simulink model "sudoku"  (R2012b)
settings: Solver=ode45  StartTime=0.0  StopTime=10.0  RelTol=1e-3
libraries: sldvlib x83
(part 2 of 4)

== system sudoku/bounds2 ==
  In1 : Inport
  Assumption : sldvlib/Objectives and Constraints/Assumption  enabled=on  customAVTBlockType=Assumption  intervals=true  initial=off  dispValues=on  outEnabled=on
      settings: AttributesFormatString=%<intervals>
  Logical Operator : Logic  AllPortsSameDT=off  OutDataTypeStr=boolean
  geq : RelationalOperator  Operator=<=  OutDataTypeStr=boolean
  lb : Constant  OutDataTypeStr=int8
  leq : RelationalOperator  Operator=<=  OutDataTypeStr=boolean
  ub : Constant  Value=9  OutDataTypeStr=int8
  wires:
  In1/1 -> geq/1, leq/2
  geq/1 -> Logical Operator/2
  ub/1 -> geq/2
  leq/1 -> Logical Operator/1
  Logical Operator/1 -> Assumption/1
  lb/1 -> leq/1

== system sudoku/bounds20 ==
  In1 : Inport
  Assumption : sldvlib/Objectives and Constraints/Assumption  enabled=on  customAVTBlockType=Assumption  intervals=true  initial=off  dispValues=on  outEnabled=on
      settings: AttributesFormatString=%<intervals>
  Logical Operator : Logic  AllPortsSameDT=off  OutDataTypeStr=boolean
  geq : RelationalOperator  Operator=<=  OutDataTypeStr=boolean
  lb : Constant  OutDataTypeStr=int8
  leq : RelationalOperator  Operator=<=  OutDataTypeStr=boolean
  ub : Constant  Value=9  OutDataTypeStr=int8
  wires:
  In1/1 -> geq/1, leq/2
  geq/1 -> Logical Operator/2
  ub/1 -> geq/2
  leq/1 -> Logical Operator/1
  Logical Operator/1 -> Assumption/1
  lb/1 -> leq/1

== system sudoku/bounds21 ==
  In1 : Inport
  Assumption : sldvlib/Objectives and Constraints/Assumption  enabled=on  customAVTBlockType=Assumption  intervals=true  initial=off  dispValues=on  outEnabled=on
      settings: AttributesFormatString=%<intervals>
  Logical Operator : Logic  AllPortsSameDT=off  OutDataTypeStr=boolean
  geq : RelationalOperator  Operator=<=  OutDataTypeStr=boolean
  lb : Constant  OutDataTypeStr=int8
  leq : RelationalOperator  Operator=<=  OutDataTypeStr=boolean
  ub : Constant  Value=9  OutDataTypeStr=int8
  wires:
  In1/1 -> geq/1, leq/2
  geq/1 -> Logical Operator/2
  ub/1 -> geq/2
  leq/1 -> Logical Operator/1
  Logical Operator/1 -> Assumption/1
  lb/1 -> leq/1

== system sudoku/bounds22 ==
  In1 : Inport
  Assumption : sldvlib/Objectives and Constraints/Assumption  enabled=on  customAVTBlockType=Assumption  intervals=true  initial=off  dispValues=on  outEnabled=on
      settings: AttributesFormatString=%<intervals>
  Logical Operator : Logic  AllPortsSameDT=off  OutDataTypeStr=boolean
  geq : RelationalOperator  Operator=<=  OutDataTypeStr=boolean
  lb : Constant  OutDataTypeStr=int8
  leq : RelationalOperator  Operator=<=  OutDataTypeStr=boolean
  ub : Constant  Value=9  OutDataTypeStr=int8
  wires:
  In1/1 -> geq/1, leq/2
  geq/1 -> Logical Operator/2
  ub/1 -> geq/2
  leq/1 -> Logical Operator/1
  Logical Operator/1 -> Assumption/1
  lb/1 -> leq/1

== system sudoku/bounds23 ==
  In1 : Inport
  Assumption : sldvlib/Objectives and Constraints/Assumption  enabled=on  customAVTBlockType=Assumption  intervals=true  initial=off  dispValues=on  outEnabled=on
      settings: AttributesFormatString=%<intervals>
  Logical Operator : Logic  AllPortsSameDT=off  OutDataTypeStr=boolean
  geq : RelationalOperator  Operator=<=  OutDataTypeStr=boolean
  lb : Constant  OutDataTypeStr=int8
  leq : RelationalOperator  Operator=<=  OutDataTypeStr=boolean
  ub : Constant  Value=9  OutDataTypeStr=int8
  wires:
  In1/1 -> geq/1, leq/2
  geq/1 -> Logical Operator/2
  ub/1 -> geq/2
  leq/1 -> Logical Operator/1
  Logical Operator/1 -> Assumption/1
  lb/1 -> leq/1

== system sudoku/bounds24 ==
  In1 : Inport
  Assumption : sldvlib/Objectives and Constraints/Assumption  enabled=on  customAVTBlockType=Assumption  intervals=true  initial=off  dispValues=on  outEnabled=on
      settings: AttributesFormatString=%<intervals>
  Logical Operator : Logic  AllPortsSameDT=off  OutDataTypeStr=boolean
  geq : RelationalOperator  Operator=<=  OutDataTypeStr=boolean
  lb : Constant  OutDataTypeStr=int8
  leq : RelationalOperator  Operator=<=  OutDataTypeStr=boolean
  ub : Constant  Value=9  OutDataTypeStr=int8
  wires:
  In1/1 -> geq/1, leq/2
  geq/1 -> Logical Operator/2
  ub/1 -> geq/2
  leq/1 -> Logical Operator/1
  Logical Operator/1 -> Assumption/1
  lb/1 -> leq/1

== system sudoku/bounds25 ==
  In1 : Inport
  Assumption : sldvlib/Objectives and Constraints/Assumption  enabled=on  customAVTBlockType=Assumption  intervals=true  initial=off  dispValues=on  outEnabled=on
      settings: AttributesFormatString=%<intervals>
  Logical Operator : Logic  AllPortsSameDT=off  OutDataTypeStr=boolean
  geq : RelationalOperator  Operator=<=  OutDataTypeStr=boolean
  lb : Constant  OutDataTypeStr=int8
  leq : RelationalOperator  Operator=<=  OutDataTypeStr=boolean
  ub : Constant  Value=9  OutDataTypeStr=int8
  wires:
  In1/1 -> geq/1, leq/2
  geq/1 -> Logical Operator/2
  ub/1 -> geq/2
  leq/1 -> Logical Operator/1
  Logical Operator/1 -> Assumption/1
  lb/1 -> leq/1

== system sudoku/bounds26 ==
  In1 : Inport
  Assumption : sldvlib/Objectives and Constraints/Assumption  enabled=on  customAVTBlockType=Assumption  intervals=true  initial=off  dispValues=on  outEnabled=on
      settings: AttributesFormatString=%<intervals>
  Logical Operator : Logic  AllPortsSameDT=off  OutDataTypeStr=boolean
  geq : RelationalOperator  Operator=<=  OutDataTypeStr=boolean
  lb : Constant  OutDataTypeStr=int8
  leq : RelationalOperator  Operator=<=  OutDataTypeStr=boolean
  ub : Constant  Value=9  OutDataTypeStr=int8
  wires:
  In1/1 -> geq/1, leq/2
  geq/1 -> Logical Operator/2
  ub/1 -> geq/2
  leq/1 -> Logical Operator/1
  Logical Operator/1 -> Assumption/1
  lb/1 -> leq/1

== system sudoku/bounds27 ==
  In1 : Inport
  Assumption : sldvlib/Objectives and Constraints/Assumption  enabled=on  customAVTBlockType=Assumption  intervals=true  initial=off  dispValues=on  outEnabled=on
      settings: AttributesFormatString=%<intervals>
  Logical Operator : Logic  AllPortsSameDT=off  OutDataTypeStr=boolean
  geq : RelationalOperator  Operator=<=  OutDataTypeStr=boolean
  lb : Constant  OutDataTypeStr=int8
  leq : RelationalOperator  Operator=<=  OutDataTypeStr=boolean
  ub : Constant  Value=9  OutDataTypeStr=int8
  wires:
  In1/1 -> geq/1, leq/2
  geq/1 -> Logical Operator/2
  ub/1 -> geq/2
  leq/1 -> Logical Operator/1
  Logical Operator/1 -> Assumption/1
  lb/1 -> leq/1

== system sudoku/bounds28 ==
  In1 : Inport
  Assumption : sldvlib/Objectives and Constraints/Assumption  enabled=on  customAVTBlockType=Assumption  intervals=true  initial=off  dispValues=on  outEnabled=on
      settings: AttributesFormatString=%<intervals>
  Logical Operator : Logic  AllPortsSameDT=off  OutDataTypeStr=boolean
  geq : RelationalOperator  Operator=<=  OutDataTypeStr=boolean
  lb : Constant  OutDataTypeStr=int8
  leq : RelationalOperator  Operator=<=  OutDataTypeStr=boolean
  ub : Constant  Value=9  OutDataTypeStr=int8
  wires:
  In1/1 -> geq/1, leq/2
  geq/1 -> Logical Operator/2
  ub/1 -> geq/2
  leq/1 -> Logical Operator/1
  Logical Operator/1 -> Assumption/1
  lb/1 -> leq/1

== system sudoku/bounds29 ==
  In1 : Inport
  Assumption : sldvlib/Objectives and Constraints/Assumption  enabled=on  customAVTBlockType=Assumption  intervals=true  initial=off  dispValues=on  outEnabled=on
      settings: AttributesFormatString=%<intervals>
  Logical Operator : Logic  AllPortsSameDT=off  OutDataTypeStr=boolean
  geq : RelationalOperator  Operator=<=  OutDataTypeStr=boolean
  lb : Constant  OutDataTypeStr=int8
  leq : RelationalOperator  Operator=<=  OutDataTypeStr=boolean
  ub : Constant  Value=9  OutDataTypeStr=int8
  wires:
  In1/1 -> geq/1, leq/2
  geq/1 -> Logical Operator/2
  ub/1 -> geq/2
  leq/1 -> Logical Operator/1
  Logical Operator/1 -> Assumption/1
  lb/1 -> leq/1

== system sudoku/bounds3 ==
  In1 : Inport
  Assumption : sldvlib/Objectives and Constraints/Assumption  enabled=on  customAVTBlockType=Assumption  intervals=true  initial=off  dispValues=on  outEnabled=on
      settings: AttributesFormatString=%<intervals>
  Logical Operator : Logic  AllPortsSameDT=off  OutDataTypeStr=boolean
  geq : RelationalOperator  Operator=<=  OutDataTypeStr=boolean
  lb : Constant  OutDataTypeStr=int8
  leq : RelationalOperator  Operator=<=  OutDataTypeStr=boolean
  ub : Constant  Value=9  OutDataTypeStr=int8
  wires:
  In1/1 -> geq/1, leq/2
  geq/1 -> Logical Operator/2
  ub/1 -> geq/2
  leq/1 -> Logical Operator/1
  Logical Operator/1 -> Assumption/1
  lb/1 -> leq/1

== system sudoku/bounds30 ==
  In1 : Inport
  Assumption : sldvlib/Objectives and Constraints/Assumption  enabled=on  customAVTBlockType=Assumption  intervals=true  initial=off  dispValues=on  outEnabled=on
      settings: AttributesFormatString=%<intervals>
  Logical Operator : Logic  AllPortsSameDT=off  OutDataTypeStr=boolean
  geq : RelationalOperator  Operator=<=  OutDataTypeStr=boolean
  lb : Constant  OutDataTypeStr=int8
  leq : RelationalOperator  Operator=<=  OutDataTypeStr=boolean
  ub : Constant  Value=9  OutDataTypeStr=int8
  wires:
  In1/1 -> geq/1, leq/2
  geq/1 -> Logical Operator/2
  ub/1 -> geq/2
  leq/1 -> Logical Operator/1
  Logical Operator/1 -> Assumption/1
  lb/1 -> leq/1

== system sudoku/bounds31 ==
  In1 : Inport
  Assumption : sldvlib/Objectives and Constraints/Assumption  enabled=on  customAVTBlockType=Assumption  intervals=true  initial=off  dispValues=on  outEnabled=on
      settings: AttributesFormatString=%<intervals>
  Logical Operator : Logic  AllPortsSameDT=off  OutDataTypeStr=boolean
  geq : RelationalOperator  Operator=<=  OutDataTypeStr=boolean
  lb : Constant  OutDataTypeStr=int8
  leq : RelationalOperator  Operator=<=  OutDataTypeStr=boolean
  ub : Constant  Value=9  OutDataTypeStr=int8
  wires:
  In1/1 -> geq/1, leq/2
  geq/1 -> Logical Operator/2
  ub/1 -> geq/2
  leq/1 -> Logical Operator/1
  Logical Operator/1 -> Assumption/1
  lb/1 -> leq/1

== system sudoku/bounds32 ==
  In1 : Inport
  Assumption : sldvlib/Objectives and Constraints/Assumption  enabled=on  customAVTBlockType=Assumption  intervals=true  initial=off  dispValues=on  outEnabled=on
      settings: AttributesFormatString=%<intervals>
  Logical Operator : Logic  AllPortsSameDT=off  OutDataTypeStr=boolean
  geq : RelationalOperator  Operator=<=  OutDataTypeStr=boolean
  lb : Constant  OutDataTypeStr=int8
  leq : RelationalOperator  Operator=<=  OutDataTypeStr=boolean
  ub : Constant  Value=9  OutDataTypeStr=int8
  wires:
  In1/1 -> geq/1, leq/2
  geq/1 -> Logical Operator/2
  ub/1 -> geq/2
  leq/1 -> Logical Operator/1
  Logical Operator/1 -> Assumption/1
  lb/1 -> leq/1

== system sudoku/bounds33 ==
  In1 : Inport
  Assumption : sldvlib/Objectives and Constraints/Assumption  enabled=on  customAVTBlockType=Assumption  intervals=true  initial=off  dispValues=on  outEnabled=on
      settings: AttributesFormatString=%<intervals>
  Logical Operator : Logic  AllPortsSameDT=off  OutDataTypeStr=boolean
  geq : RelationalOperator  Operator=<=  OutDataTypeStr=boolean
  lb : Constant  OutDataTypeStr=int8
  leq : RelationalOperator  Operator=<=  OutDataTypeStr=boolean
  ub : Constant  Value=9  OutDataTypeStr=int8
  wires:
  In1/1 -> geq/1, leq/2
  geq/1 -> Logical Operator/2
  ub/1 -> geq/2
  leq/1 -> Logical Operator/1
  Logical Operator/1 -> Assumption/1
  lb/1 -> leq/1

== system sudoku/bounds34 ==
  In1 : Inport
  Assumption : sldvlib/Objectives and Constraints/Assumption  enabled=on  customAVTBlockType=Assumption  intervals=true  initial=off  dispValues=on  outEnabled=on
      settings: AttributesFormatString=%<intervals>
  Logical Operator : Logic  AllPortsSameDT=off  OutDataTypeStr=boolean
  geq : RelationalOperator  Operator=<=  OutDataTypeStr=boolean
  lb : Constant  OutDataTypeStr=int8
  leq : RelationalOperator  Operator=<=  OutDataTypeStr=boolean
  ub : Constant  Value=9  OutDataTypeStr=int8
  wires:
  In1/1 -> geq/1, leq/2
  geq/1 -> Logical Operator/2
  ub/1 -> geq/2
  leq/1 -> Logical Operator/1
  Logical Operator/1 -> Assumption/1
  lb/1 -> leq/1

== system sudoku/bounds35 ==
  In1 : Inport
  Assumption : sldvlib/Objectives and Constraints/Assumption  enabled=on  customAVTBlockType=Assumption  intervals=true  initial=off  dispValues=on  outEnabled=on
      settings: AttributesFormatString=%<intervals>
  Logical Operator : Logic  AllPortsSameDT=off  OutDataTypeStr=boolean
  geq : RelationalOperator  Operator=<=  OutDataTypeStr=boolean
  lb : Constant  OutDataTypeStr=int8
  leq : RelationalOperator  Operator=<=  OutDataTypeStr=boolean
  ub : Constant  Value=9  OutDataTypeStr=int8
  wires:
  In1/1 -> geq/1, leq/2
  geq/1 -> Logical Operator/2
  ub/1 -> geq/2
  leq/1 -> Logical Operator/1
  Logical Operator/1 -> Assumption/1
  lb/1 -> leq/1

== system sudoku/bounds36 ==
  In1 : Inport
  Assumption : sldvlib/Objectives and Constraints/Assumption  enabled=on  customAVTBlockType=Assumption  intervals=true  initial=off  dispValues=on  outEnabled=on
      settings: AttributesFormatString=%<intervals>
  Logical Operator : Logic  AllPortsSameDT=off  OutDataTypeStr=boolean
  geq : RelationalOperator  Operator=<=  OutDataTypeStr=boolean
  lb : Constant  OutDataTypeStr=int8
  leq : RelationalOperator  Operator=<=  OutDataTypeStr=boolean
  ub : Constant  Value=9  OutDataTypeStr=int8
  wires:
  In1/1 -> geq/1, leq/2
  geq/1 -> Logical Operator/2
  ub/1 -> geq/2
  leq/1 -> Logical Operator/1
  Logical Operator/1 -> Assumption/1
  lb/1 -> leq/1

== system sudoku/bounds37 ==
  In1 : Inport
  Assumption : sldvlib/Objectives and Constraints/Assumption  enabled=on  customAVTBlockType=Assumption  intervals=true  initial=off  dispValues=on  outEnabled=on
      settings: AttributesFormatString=%<intervals>
  Logical Operator : Logic  AllPortsSameDT=off  OutDataTypeStr=boolean
  geq : RelationalOperator  Operator=<=  OutDataTypeStr=boolean
  lb : Constant  OutDataTypeStr=int8
  leq : RelationalOperator  Operator=<=  OutDataTypeStr=boolean
  ub : Constant  Value=9  OutDataTypeStr=int8
  wires:
  In1/1 -> geq/1, leq/2
  geq/1 -> Logical Operator/2
  ub/1 -> geq/2
  leq/1 -> Logical Operator/1
  Logical Operator/1 -> Assumption/1
  lb/1 -> leq/1

== system sudoku/bounds38 ==
  In1 : Inport
  Assumption : sldvlib/Objectives and Constraints/Assumption  enabled=on  customAVTBlockType=Assumption  intervals=true  initial=off  dispValues=on  outEnabled=on
      settings: AttributesFormatString=%<intervals>
  Logical Operator : Logic  AllPortsSameDT=off  OutDataTypeStr=boolean
  geq : RelationalOperator  Operator=<=  OutDataTypeStr=boolean
  lb : Constant  OutDataTypeStr=int8
  leq : RelationalOperator  Operator=<=  OutDataTypeStr=boolean
  ub : Constant  Value=9  OutDataTypeStr=int8
  wires:
  In1/1 -> geq/1, leq/2
  geq/1 -> Logical Operator/2
  ub/1 -> geq/2
  leq/1 -> Logical Operator/1
  Logical Operator/1 -> Assumption/1
  lb/1 -> leq/1

== system sudoku/bounds39 ==
  In1 : Inport
  Assumption : sldvlib/Objectives and Constraints/Assumption  enabled=on  customAVTBlockType=Assumption  intervals=true  initial=off  dispValues=on  outEnabled=on
      settings: AttributesFormatString=%<intervals>
  Logical Operator : Logic  AllPortsSameDT=off  OutDataTypeStr=boolean
  geq : RelationalOperator  Operator=<=  OutDataTypeStr=boolean
  lb : Constant  OutDataTypeStr=int8
  leq : RelationalOperator  Operator=<=  OutDataTypeStr=boolean
  ub : Constant  Value=9  OutDataTypeStr=int8
  wires:
  In1/1 -> geq/1, leq/2
  geq/1 -> Logical Operator/2
  ub/1 -> geq/2
  leq/1 -> Logical Operator/1
  Logical Operator/1 -> Assumption/1
  lb/1 -> leq/1

== system sudoku/bounds4 ==
  In1 : Inport
  Assumption : sldvlib/Objectives and Constraints/Assumption  enabled=on  customAVTBlockType=Assumption  intervals=true  initial=off  dispValues=on  outEnabled=on
      settings: AttributesFormatString=%<intervals>
  Logical Operator : Logic  AllPortsSameDT=off  OutDataTypeStr=boolean
  geq : RelationalOperator  Operator=<=  OutDataTypeStr=boolean
  lb : Constant  OutDataTypeStr=int8
  leq : RelationalOperator  Operator=<=  OutDataTypeStr=boolean
  ub : Constant  Value=9  OutDataTypeStr=int8
  wires:
  In1/1 -> geq/1, leq/2
  geq/1 -> Logical Operator/2
  ub/1 -> geq/2
  leq/1 -> Logical Operator/1
  Logical Operator/1 -> Assumption/1
  lb/1 -> leq/1

== system sudoku/bounds40 ==
  In1 : Inport
  Assumption : sldvlib/Objectives and Constraints/Assumption  enabled=on  customAVTBlockType=Assumption  intervals=true  initial=off  dispValues=on  outEnabled=on
      settings: AttributesFormatString=%<intervals>
  Logical Operator : Logic  AllPortsSameDT=off  OutDataTypeStr=boolean
  geq : RelationalOperator  Operator=<=  OutDataTypeStr=boolean
  lb : Constant  OutDataTypeStr=int8
  leq : RelationalOperator  Operator=<=  OutDataTypeStr=boolean
  ub : Constant  Value=9  OutDataTypeStr=int8
  wires:
  In1/1 -> geq/1, leq/2
  geq/1 -> Logical Operator/2
  ub/1 -> geq/2
  leq/1 -> Logical Operator/1
  Logical Operator/1 -> Assumption/1
  lb/1 -> leq/1

== system sudoku/bounds41 ==
  In1 : Inport
  Assumption : sldvlib/Objectives and Constraints/Assumption  enabled=on  customAVTBlockType=Assumption  intervals=true  initial=off  dispValues=on  outEnabled=on
      settings: AttributesFormatString=%<intervals>
  Logical Operator : Logic  AllPortsSameDT=off  OutDataTypeStr=boolean
  geq : RelationalOperator  Operator=<=  OutDataTypeStr=boolean
  lb : Constant  OutDataTypeStr=int8
  leq : RelationalOperator  Operator=<=  OutDataTypeStr=boolean  InputSameDT=on
  ub : Constant  Value=9  OutDataTypeStr=int8
  wires:
  In1/1 -> geq/1, leq/2
  geq/1 -> Logical Operator/2
  ub/1 -> geq/2
  leq/1 -> Logical Operator/1
  Logical Operator/1 -> Assumption/1
  lb/1 -> leq/1

== system sudoku/bounds42 ==
  In1 : Inport
  Assumption : sldvlib/Objectives and Constraints/Assumption  enabled=on  customAVTBlockType=Assumption  intervals=true  initial=off  dispValues=on  outEnabled=on
      settings: AttributesFormatString=%<intervals>
  Logical Operator : Logic  AllPortsSameDT=off  OutDataTypeStr=boolean
  geq : RelationalOperator  Operator=<=  OutDataTypeStr=boolean
  lb : Constant  OutDataTypeStr=int8
  leq : RelationalOperator  Operator=<=  OutDataTypeStr=boolean  InputSameDT=on
  ub : Constant  Value=9  OutDataTypeStr=int8
  wires:
  In1/1 -> geq/1, leq/2
  geq/1 -> Logical Operator/2
  ub/1 -> geq/2
  leq/1 -> Logical Operator/1
  Logical Operator/1 -> Assumption/1
  lb/1 -> leq/1

== system sudoku/bounds43 ==
  In1 : Inport
  Assumption : sldvlib/Objectives and Constraints/Assumption  enabled=on  customAVTBlockType=Assumption  intervals=true  initial=off  dispValues=on  outEnabled=on
      settings: AttributesFormatString=%<intervals>
  Logical Operator : Logic  AllPortsSameDT=off  OutDataTypeStr=boolean
  geq : RelationalOperator  Operator=<=  OutDataTypeStr=boolean
  lb : Constant  OutDataTypeStr=int8
  leq : RelationalOperator  Operator=<=  OutDataTypeStr=boolean  InputSameDT=on
  ub : Constant  Value=9  OutDataTypeStr=int8
  wires:
  In1/1 -> geq/1, leq/2
  geq/1 -> Logical Operator/2
  ub/1 -> geq/2
  leq/1 -> Logical Operator/1
  Logical Operator/1 -> Assumption/1
  lb/1 -> leq/1

== system sudoku/bounds44 ==
  In1 : Inport
  Assumption : sldvlib/Objectives and Constraints/Assumption  enabled=on  customAVTBlockType=Assumption  intervals=true  initial=off  dispValues=on  outEnabled=on
      settings: AttributesFormatString=%<intervals>
  Logical Operator : Logic  AllPortsSameDT=off  OutDataTypeStr=boolean
  geq : RelationalOperator  Operator=<=  OutDataTypeStr=boolean
  lb : Constant  OutDataTypeStr=int8
  leq : RelationalOperator  Operator=<=  OutDataTypeStr=boolean  InputSameDT=on
  ub : Constant  Value=9  OutDataTypeStr=int8
  wires:
  In1/1 -> geq/1, leq/2
  geq/1 -> Logical Operator/2
  ub/1 -> geq/2
  leq/1 -> Logical Operator/1
  Logical Operator/1 -> Assumption/1
  lb/1 -> leq/1

== system sudoku/bounds45 ==
  In1 : Inport
  Assumption : sldvlib/Objectives and Constraints/Assumption  enabled=on  customAVTBlockType=Assumption  intervals=true  initial=off  dispValues=on  outEnabled=on
      settings: AttributesFormatString=%<intervals>
  Logical Operator : Logic  AllPortsSameDT=off  OutDataTypeStr=boolean
  geq : RelationalOperator  Operator=<=  OutDataTypeStr=boolean
  lb : Constant  OutDataTypeStr=int8
  leq : RelationalOperator  Operator=<=  OutDataTypeStr=boolean  InputSameDT=on
  ub : Constant  Value=9  OutDataTypeStr=int8
  wires:
  In1/1 -> geq/1, leq/2
  geq/1 -> Logical Operator/2
  ub/1 -> geq/2
  leq/1 -> Logical Operator/1
  Logical Operator/1 -> Assumption/1
  lb/1 -> leq/1

== system sudoku/bounds46 ==
  In1 : Inport
  Assumption : sldvlib/Objectives and Constraints/Assumption  enabled=on  customAVTBlockType=Assumption  intervals=true  initial=off  dispValues=on  outEnabled=on
      settings: AttributesFormatString=%<intervals>
  Logical Operator : Logic  AllPortsSameDT=off  OutDataTypeStr=boolean
  geq : RelationalOperator  Operator=<=  OutDataTypeStr=boolean
  lb : Constant  OutDataTypeStr=int8
  leq : RelationalOperator  Operator=<=  OutDataTypeStr=boolean  InputSameDT=on
  ub : Constant  Value=9  OutDataTypeStr=int8
  wires:
  In1/1 -> geq/1, leq/2
  geq/1 -> Logical Operator/2
  ub/1 -> geq/2
  leq/1 -> Logical Operator/1
  Logical Operator/1 -> Assumption/1
  lb/1 -> leq/1

== system sudoku/bounds47 ==
  In1 : Inport
  Assumption : sldvlib/Objectives and Constraints/Assumption  enabled=on  customAVTBlockType=Assumption  intervals=true  initial=off  dispValues=on  outEnabled=on
      settings: AttributesFormatString=%<intervals>
  Logical Operator : Logic  AllPortsSameDT=off  OutDataTypeStr=boolean
  geq : RelationalOperator  Operator=<=  OutDataTypeStr=boolean
  lb : Constant  OutDataTypeStr=int8
  leq : RelationalOperator  Operator=<=  OutDataTypeStr=boolean  InputSameDT=on
  ub : Constant  Value=9  OutDataTypeStr=int8
  wires:
  In1/1 -> geq/1, leq/2
  geq/1 -> Logical Operator/2
  ub/1 -> geq/2
  leq/1 -> Logical Operator/1
  Logical Operator/1 -> Assumption/1
  lb/1 -> leq/1

== system sudoku/bounds48 ==
  In1 : Inport
  Assumption : sldvlib/Objectives and Constraints/Assumption  enabled=on  customAVTBlockType=Assumption  intervals=true  initial=off  dispValues=on  outEnabled=on
      settings: AttributesFormatString=%<intervals>
  Logical Operator : Logic  AllPortsSameDT=off  OutDataTypeStr=boolean
  geq : RelationalOperator  Operator=<=  OutDataTypeStr=boolean
  lb : Constant  OutDataTypeStr=int8
  leq : RelationalOperator  Operator=<=  OutDataTypeStr=boolean  InputSameDT=on
  ub : Constant  Value=9  OutDataTypeStr=int8
  wires:
  In1/1 -> geq/1, leq/2
  geq/1 -> Logical Operator/2
  ub/1 -> geq/2
  leq/1 -> Logical Operator/1
  Logical Operator/1 -> Assumption/1
  lb/1 -> leq/1

== system sudoku/bounds49 ==
  In1 : Inport
  Assumption : sldvlib/Objectives and Constraints/Assumption  enabled=on  customAVTBlockType=Assumption  intervals=true  initial=off  dispValues=on  outEnabled=on
      settings: AttributesFormatString=%<intervals>
  Logical Operator : Logic  AllPortsSameDT=off  OutDataTypeStr=boolean
  geq : RelationalOperator  Operator=<=  OutDataTypeStr=boolean
  lb : Constant  OutDataTypeStr=int8
  leq : RelationalOperator  Operator=<=  OutDataTypeStr=boolean  InputSameDT=on
  ub : Constant  Value=9  OutDataTypeStr=int8
  wires:
  In1/1 -> geq/1, leq/2
  geq/1 -> Logical Operator/2
  ub/1 -> geq/2
  leq/1 -> Logical Operator/1
  Logical Operator/1 -> Assumption/1
  lb/1 -> leq/1

== system sudoku/bounds5 ==
  In1 : Inport
  Assumption : sldvlib/Objectives and Constraints/Assumption  enabled=on  customAVTBlockType=Assumption  intervals=true  initial=off  dispValues=on  outEnabled=on
      settings: AttributesFormatString=%<intervals>
  Logical Operator : Logic  AllPortsSameDT=off  OutDataTypeStr=boolean
  geq : RelationalOperator  Operator=<=  OutDataTypeStr=boolean
  lb : Constant  OutDataTypeStr=int8
  leq : RelationalOperator  Operator=<=  OutDataTypeStr=boolean
  ub : Constant  Value=9  OutDataTypeStr=int8
  wires:
  In1/1 -> geq/1, leq/2
  geq/1 -> Logical Operator/2
  ub/1 -> geq/2
  leq/1 -> Logical Operator/1
  Logical Operator/1 -> Assumption/1
  lb/1 -> leq/1

== system sudoku/bounds50 ==
  In1 : Inport
  Assumption : sldvlib/Objectives and Constraints/Assumption  enabled=on  customAVTBlockType=Assumption  intervals=true  initial=off  dispValues=on  outEnabled=on
      settings: AttributesFormatString=%<intervals>
  Logical Operator : Logic  AllPortsSameDT=off  OutDataTypeStr=boolean
  geq : RelationalOperator  Operator=<=  OutDataTypeStr=boolean
  lb : Constant  OutDataTypeStr=int8
  leq : RelationalOperator  Operator=<=  OutDataTypeStr=boolean  InputSameDT=on
  ub : Constant  Value=9  OutDataTypeStr=int8
  wires:
  In1/1 -> geq/1, leq/2
  geq/1 -> Logical Operator/2
  ub/1 -> geq/2
  leq/1 -> Logical Operator/1
  Logical Operator/1 -> Assumption/1
  lb/1 -> leq/1

== system sudoku/bounds51 ==
  In1 : Inport
  Assumption : sldvlib/Objectives and Constraints/Assumption  enabled=on  customAVTBlockType=Assumption  intervals=true  initial=off  dispValues=on  outEnabled=on
      settings: AttributesFormatString=%<intervals>
  Logical Operator : Logic  AllPortsSameDT=off  OutDataTypeStr=boolean
  geq : RelationalOperator  Operator=<=  OutDataTypeStr=boolean
  lb : Constant  OutDataTypeStr=int8
  leq : RelationalOperator  Operator=<=  OutDataTypeStr=boolean  InputSameDT=on
  ub : Constant  Value=9  OutDataTypeStr=int8
  wires:
  In1/1 -> geq/1, leq/2
  geq/1 -> Logical Operator/2
  ub/1 -> geq/2
  leq/1 -> Logical Operator/1
  Logical Operator/1 -> Assumption/1
  lb/1 -> leq/1

== system sudoku/bounds52 ==
  In1 : Inport
  Assumption : sldvlib/Objectives and Constraints/Assumption  enabled=on  customAVTBlockType=Assumption  intervals=true  initial=off  dispValues=on  outEnabled=on
      settings: AttributesFormatString=%<intervals>
  Logical Operator : Logic  AllPortsSameDT=off  OutDataTypeStr=boolean
  geq : RelationalOperator  Operator=<=  OutDataTypeStr=boolean
  lb : Constant  OutDataTypeStr=int8
  leq : RelationalOperator  Operator=<=  OutDataTypeStr=boolean  InputSameDT=on
  ub : Constant  Value=9  OutDataTypeStr=int8
  wires:
  In1/1 -> geq/1, leq/2
  geq/1 -> Logical Operator/2
  ub/1 -> geq/2
  leq/1 -> Logical Operator/1
  Logical Operator/1 -> Assumption/1
  lb/1 -> leq/1

== system sudoku/bounds53 ==
  In1 : Inport
  Assumption : sldvlib/Objectives and Constraints/Assumption  enabled=on  customAVTBlockType=Assumption  intervals=true  initial=off  dispValues=on  outEnabled=on
      settings: AttributesFormatString=%<intervals>
  Logical Operator : Logic  AllPortsSameDT=off  OutDataTypeStr=boolean
  geq : RelationalOperator  Operator=<=  OutDataTypeStr=boolean
  lb : Constant  OutDataTypeStr=int8
  leq : RelationalOperator  Operator=<=  OutDataTypeStr=boolean  InputSameDT=on
  ub : Constant  Value=9  OutDataTypeStr=int8
  wires:
  In1/1 -> geq/1, leq/2
  geq/1 -> Logical Operator/2
  ub/1 -> geq/2
  leq/1 -> Logical Operator/1
  Logical Operator/1 -> Assumption/1
  lb/1 -> leq/1

== system sudoku/bounds54 ==
  In1 : Inport
  Assumption : sldvlib/Objectives and Constraints/Assumption  enabled=on  customAVTBlockType=Assumption  intervals=true  initial=off  dispValues=on  outEnabled=on
      settings: AttributesFormatString=%<intervals>
  Logical Operator : Logic  AllPortsSameDT=off  OutDataTypeStr=boolean
  geq : RelationalOperator  Operator=<=  OutDataTypeStr=boolean
  lb : Constant  OutDataTypeStr=int8
  leq : RelationalOperator  Operator=<=  OutDataTypeStr=boolean  InputSameDT=on
  ub : Constant  Value=9  OutDataTypeStr=int8
  wires:
  In1/1 -> geq/1, leq/2
  geq/1 -> Logical Operator/2
  ub/1 -> geq/2
  leq/1 -> Logical Operator/1
  Logical Operator/1 -> Assumption/1
  lb/1 -> leq/1

== system sudoku/bounds55 ==
  In1 : Inport
  Assumption : sldvlib/Objectives and Constraints/Assumption  enabled=on  customAVTBlockType=Assumption  intervals=true  initial=off  dispValues=on  outEnabled=on
      settings: AttributesFormatString=%<intervals>
  Logical Operator : Logic  AllPortsSameDT=off  OutDataTypeStr=boolean
  geq : RelationalOperator  Operator=<=  OutDataTypeStr=boolean
  lb : Constant  OutDataTypeStr=int8
  leq : RelationalOperator  Operator=<=  OutDataTypeStr=boolean  InputSameDT=on
  ub : Constant  Value=9  OutDataTypeStr=int8
  wires:
  In1/1 -> geq/1, leq/2
  geq/1 -> Logical Operator/2
  ub/1 -> geq/2
  leq/1 -> Logical Operator/1
  Logical Operator/1 -> Assumption/1
  lb/1 -> leq/1

== system sudoku/bounds56 ==
  In1 : Inport
  Assumption : sldvlib/Objectives and Constraints/Assumption  enabled=on  customAVTBlockType=Assumption  intervals=true  initial=off  dispValues=on  outEnabled=on
      settings: AttributesFormatString=%<intervals>
  Logical Operator : Logic  AllPortsSameDT=off  OutDataTypeStr=boolean
  geq : RelationalOperator  Operator=<=  OutDataTypeStr=boolean
  lb : Constant  OutDataTypeStr=int8
  leq : RelationalOperator  Operator=<=  OutDataTypeStr=boolean  InputSameDT=on
  ub : Constant  Value=9  OutDataTypeStr=int8
  wires:
  In1/1 -> geq/1, leq/2
  geq/1 -> Logical Operator/2
  ub/1 -> geq/2
  leq/1 -> Logical Operator/1
  Logical Operator/1 -> Assumption/1
  lb/1 -> leq/1

== system sudoku/bounds57 ==
  In1 : Inport
  Assumption : sldvlib/Objectives and Constraints/Assumption  enabled=on  customAVTBlockType=Assumption  intervals=true  initial=off  dispValues=on  outEnabled=on
      settings: AttributesFormatString=%<intervals>
  Logical Operator : Logic  AllPortsSameDT=off  OutDataTypeStr=boolean
  geq : RelationalOperator  Operator=<=  OutDataTypeStr=boolean
  lb : Constant  OutDataTypeStr=int8
  leq : RelationalOperator  Operator=<=  OutDataTypeStr=boolean  InputSameDT=on
  ub : Constant  Value=9  OutDataTypeStr=int8
  wires:
  In1/1 -> geq/1, leq/2
  geq/1 -> Logical Operator/2
  ub/1 -> geq/2
  leq/1 -> Logical Operator/1
  Logical Operator/1 -> Assumption/1
  lb/1 -> leq/1

== system sudoku/bounds58 ==
  In1 : Inport
  Assumption : sldvlib/Objectives and Constraints/Assumption  enabled=on  customAVTBlockType=Assumption  intervals=true  initial=off  dispValues=on  outEnabled=on
      settings: AttributesFormatString=%<intervals>
  Logical Operator : Logic  AllPortsSameDT=off  OutDataTypeStr=boolean
  geq : RelationalOperator  Operator=<=  OutDataTypeStr=boolean
  lb : Constant  OutDataTypeStr=int8
  leq : RelationalOperator  Operator=<=  OutDataTypeStr=boolean  InputSameDT=on
  ub : Constant  Value=9  OutDataTypeStr=int8
  wires:
  In1/1 -> geq/1, leq/2
  geq/1 -> Logical Operator/2
  ub/1 -> geq/2
  leq/1 -> Logical Operator/1
  Logical Operator/1 -> Assumption/1
  lb/1 -> leq/1

== system sudoku/bounds59 ==
  In1 : Inport
  Assumption : sldvlib/Objectives and Constraints/Assumption  enabled=on  customAVTBlockType=Assumption  intervals=true  initial=off  dispValues=on  outEnabled=on
      settings: AttributesFormatString=%<intervals>
  Logical Operator : Logic  AllPortsSameDT=off  OutDataTypeStr=boolean
  geq : RelationalOperator  Operator=<=  OutDataTypeStr=boolean
  lb : Constant  OutDataTypeStr=int8
  leq : RelationalOperator  Operator=<=  OutDataTypeStr=boolean  InputSameDT=on
  ub : Constant  Value=9  OutDataTypeStr=int8
  wires:
  In1/1 -> geq/1, leq/2
  geq/1 -> Logical Operator/2
  ub/1 -> geq/2
  leq/1 -> Logical Operator/1
  Logical Operator/1 -> Assumption/1
  lb/1 -> leq/1

== system sudoku/bounds6 ==
  In1 : Inport
  Assumption : sldvlib/Objectives and Constraints/Assumption  enabled=on  customAVTBlockType=Assumption  intervals=true  initial=off  dispValues=on  outEnabled=on
      settings: AttributesFormatString=%<intervals>
  Logical Operator : Logic  AllPortsSameDT=off  OutDataTypeStr=boolean
  geq : RelationalOperator  Operator=<=  OutDataTypeStr=boolean
  lb : Constant  OutDataTypeStr=int8
  leq : RelationalOperator  Operator=<=  OutDataTypeStr=boolean
  ub : Constant  Value=9  OutDataTypeStr=int8
  wires:
  In1/1 -> geq/1, leq/2
  geq/1 -> Logical Operator/2
  ub/1 -> geq/2
  leq/1 -> Logical Operator/1
  Logical Operator/1 -> Assumption/1
  lb/1 -> leq/1

== system sudoku/bounds60 ==
  In1 : Inport
  Assumption : sldvlib/Objectives and Constraints/Assumption  enabled=on  customAVTBlockType=Assumption  intervals=true  initial=off  dispValues=on  outEnabled=on
      settings: AttributesFormatString=%<intervals>
  Logical Operator : Logic  AllPortsSameDT=off  OutDataTypeStr=boolean
  geq : RelationalOperator  Operator=<=  OutDataTypeStr=boolean
  lb : Constant  OutDataTypeStr=int8
  leq : RelationalOperator  Operator=<=  OutDataTypeStr=boolean  InputSameDT=on
  ub : Constant  Value=9  OutDataTypeStr=int8
  wires:
  In1/1 -> geq/1, leq/2
  geq/1 -> Logical Operator/2
  ub/1 -> geq/2
  leq/1 -> Logical Operator/1
  Logical Operator/1 -> Assumption/1
  lb/1 -> leq/1

== system sudoku/bounds61 ==
  In1 : Inport
  Assumption : sldvlib/Objectives and Constraints/Assumption  enabled=on  customAVTBlockType=Assumption  intervals=true  initial=off  dispValues=on  outEnabled=on
      settings: AttributesFormatString=%<intervals>
  Logical Operator : Logic  AllPortsSameDT=off  OutDataTypeStr=boolean
  geq : RelationalOperator  Operator=<=  OutDataTypeStr=boolean
  lb : Constant  OutDataTypeStr=int8
  leq : RelationalOperator  Operator=<=  OutDataTypeStr=boolean  InputSameDT=on
  ub : Constant  Value=9  OutDataTypeStr=int8
  wires:
  In1/1 -> geq/1, leq/2
  geq/1 -> Logical Operator/2
  ub/1 -> geq/2
  leq/1 -> Logical Operator/1
  Logical Operator/1 -> Assumption/1
  lb/1 -> leq/1

== system sudoku/bounds62 ==
  In1 : Inport
  Assumption : sldvlib/Objectives and Constraints/Assumption  enabled=on  customAVTBlockType=Assumption  intervals=true  initial=off  dispValues=on  outEnabled=on
      settings: AttributesFormatString=%<intervals>
  Logical Operator : Logic  AllPortsSameDT=off  OutDataTypeStr=boolean
  geq : RelationalOperator  Operator=<=  OutDataTypeStr=boolean
  lb : Constant  OutDataTypeStr=int8
  leq : RelationalOperator  Operator=<=  OutDataTypeStr=boolean  InputSameDT=on
  ub : Constant  Value=9  OutDataTypeStr=int8
  wires:
  In1/1 -> geq/1, leq/2
  geq/1 -> Logical Operator/2
  ub/1 -> geq/2
  leq/1 -> Logical Operator/1
  Logical Operator/1 -> Assumption/1
  lb/1 -> leq/1

== system sudoku/bounds63 ==
  In1 : Inport
  Assumption : sldvlib/Objectives and Constraints/Assumption  enabled=on  customAVTBlockType=Assumption  intervals=true  initial=off  dispValues=on  outEnabled=on
      settings: AttributesFormatString=%<intervals>
  Logical Operator : Logic  AllPortsSameDT=off  OutDataTypeStr=boolean
  geq : RelationalOperator  Operator=<=  OutDataTypeStr=boolean
  lb : Constant  OutDataTypeStr=int8
  leq : RelationalOperator  Operator=<=  OutDataTypeStr=boolean  InputSameDT=on
  ub : Constant  Value=9  OutDataTypeStr=int8
  wires:
  In1/1 -> geq/1, leq/2
  geq/1 -> Logical Operator/2
  ub/1 -> geq/2
  leq/1 -> Logical Operator/1
  Logical Operator/1 -> Assumption/1
  lb/1 -> leq/1

== system sudoku/bounds64 ==
  In1 : Inport
  Assumption : sldvlib/Objectives and Constraints/Assumption  enabled=on  customAVTBlockType=Assumption  intervals=true  initial=off  dispValues=on  outEnabled=on
      settings: AttributesFormatString=%<intervals>
  Logical Operator : Logic  AllPortsSameDT=off  OutDataTypeStr=boolean
  geq : RelationalOperator  Operator=<=  OutDataTypeStr=boolean
  lb : Constant  OutDataTypeStr=int8
  leq : RelationalOperator  Operator=<=  OutDataTypeStr=boolean  InputSameDT=on
  ub : Constant  Value=9  OutDataTypeStr=int8
  wires:
  In1/1 -> geq/1, leq/2
  geq/1 -> Logical Operator/2
  ub/1 -> geq/2
  leq/1 -> Logical Operator/1
  Logical Operator/1 -> Assumption/1
  lb/1 -> leq/1

== system sudoku/bounds65 ==
  In1 : Inport
  Assumption : sldvlib/Objectives and Constraints/Assumption  enabled=on  customAVTBlockType=Assumption  intervals=true  initial=off  dispValues=on  outEnabled=on
      settings: AttributesFormatString=%<intervals>
  Logical Operator : Logic  AllPortsSameDT=off  OutDataTypeStr=boolean
  geq : RelationalOperator  Operator=<=  OutDataTypeStr=boolean
  lb : Constant  OutDataTypeStr=int8
  leq : RelationalOperator  Operator=<=  OutDataTypeStr=boolean  InputSameDT=on
  ub : Constant  Value=9  OutDataTypeStr=int8
  wires:
  In1/1 -> geq/1, leq/2
  geq/1 -> Logical Operator/2
  ub/1 -> geq/2
  leq/1 -> Logical Operator/1
  Logical Operator/1 -> Assumption/1
  lb/1 -> leq/1

== system sudoku/bounds66 ==
  In1 : Inport
  Assumption : sldvlib/Objectives and Constraints/Assumption  enabled=on  customAVTBlockType=Assumption  intervals=true  initial=off  dispValues=on  outEnabled=on
      settings: AttributesFormatString=%<intervals>
  Logical Operator : Logic  AllPortsSameDT=off  OutDataTypeStr=boolean
  geq : RelationalOperator  Operator=<=  OutDataTypeStr=boolean
  lb : Constant  OutDataTypeStr=int8
  leq : RelationalOperator  Operator=<=  OutDataTypeStr=boolean  InputSameDT=on
  ub : Constant  Value=9  OutDataTypeStr=int8
  wires:
  In1/1 -> geq/1, leq/2
  geq/1 -> Logical Operator/2
  ub/1 -> geq/2
  leq/1 -> Logical Operator/1
  Logical Operator/1 -> Assumption/1
  lb/1 -> leq/1

== system sudoku/bounds67 ==
  In1 : Inport
  Assumption : sldvlib/Objectives and Constraints/Assumption  enabled=on  customAVTBlockType=Assumption  intervals=true  initial=off  dispValues=on  outEnabled=on
      settings: AttributesFormatString=%<intervals>
  Logical Operator : Logic  AllPortsSameDT=off  OutDataTypeStr=boolean
  geq : RelationalOperator  Operator=<=  OutDataTypeStr=boolean
  lb : Constant  OutDataTypeStr=int8
  leq : RelationalOperator  Operator=<=  OutDataTypeStr=boolean  InputSameDT=on
  ub : Constant  Value=9  OutDataTypeStr=int8
  wires:
  In1/1 -> geq/1, leq/2
  geq/1 -> Logical Operator/2
  ub/1 -> geq/2
  leq/1 -> Logical Operator/1
  Logical Operator/1 -> Assumption/1
  lb/1 -> leq/1

== system sudoku/bounds68 ==
  In1 : Inport
  Assumption : sldvlib/Objectives and Constraints/Assumption  enabled=on  customAVTBlockType=Assumption  intervals=true  initial=off  dispValues=on  outEnabled=on
      settings: AttributesFormatString=%<intervals>
  Logical Operator : Logic  AllPortsSameDT=off  OutDataTypeStr=boolean
  geq : RelationalOperator  Operator=<=  OutDataTypeStr=boolean
  lb : Constant  OutDataTypeStr=int8
  leq : RelationalOperator  Operator=<=  OutDataTypeStr=boolean  InputSameDT=on
  ub : Constant  Value=9  OutDataTypeStr=int8
  wires:
  In1/1 -> geq/1, leq/2
  geq/1 -> Logical Operator/2
  ub/1 -> geq/2
  leq/1 -> Logical Operator/1
  Logical Operator/1 -> Assumption/1
  lb/1 -> leq/1

== system sudoku/bounds69 ==
  In1 : Inport
  Assumption : sldvlib/Objectives and Constraints/Assumption  enabled=on  customAVTBlockType=Assumption  intervals=true  initial=off  dispValues=on  outEnabled=on
      settings: AttributesFormatString=%<intervals>
  Logical Operator : Logic  AllPortsSameDT=off  OutDataTypeStr=boolean
  geq : RelationalOperator  Operator=<=  OutDataTypeStr=boolean
  lb : Constant  OutDataTypeStr=int8
  leq : RelationalOperator  Operator=<=  OutDataTypeStr=boolean  InputSameDT=on
  ub : Constant  Value=9  OutDataTypeStr=int8
  wires:
  In1/1 -> geq/1, leq/2
  geq/1 -> Logical Operator/2
  ub/1 -> geq/2
  leq/1 -> Logical Operator/1
  Logical Operator/1 -> Assumption/1
  lb/1 -> leq/1

== system sudoku/bounds7 ==
  In1 : Inport
  Assumption : sldvlib/Objectives and Constraints/Assumption  enabled=on  customAVTBlockType=Assumption  intervals=true  initial=off  dispValues=on  outEnabled=on
      settings: AttributesFormatString=%<intervals>
  Logical Operator : Logic  AllPortsSameDT=off  OutDataTypeStr=boolean
  geq : RelationalOperator  Operator=<=  OutDataTypeStr=boolean
  lb : Constant  OutDataTypeStr=int8
  leq : RelationalOperator  Operator=<=  OutDataTypeStr=boolean
  ub : Constant  Value=9  OutDataTypeStr=int8
  wires:
  In1/1 -> geq/1, leq/2
  geq/1 -> Logical Operator/2
  ub/1 -> geq/2
  leq/1 -> Logical Operator/1
  Logical Operator/1 -> Assumption/1
  lb/1 -> leq/1

== system sudoku/bounds70 ==
  In1 : Inport
  Assumption : sldvlib/Objectives and Constraints/Assumption  enabled=on  customAVTBlockType=Assumption  intervals=true  initial=off  dispValues=on  outEnabled=on
      settings: AttributesFormatString=%<intervals>
  Logical Operator : Logic  AllPortsSameDT=off  OutDataTypeStr=boolean
  geq : RelationalOperator  Operator=<=  OutDataTypeStr=boolean
  lb : Constant  OutDataTypeStr=int8
  leq : RelationalOperator  Operator=<=  OutDataTypeStr=boolean  InputSameDT=on
  ub : Constant  Value=9  OutDataTypeStr=int8
  wires:
  In1/1 -> geq/1, leq/2
  geq/1 -> Logical Operator/2
  ub/1 -> geq/2
  leq/1 -> Logical Operator/1
  Logical Operator/1 -> Assumption/1
  lb/1 -> leq/1

== system sudoku/bounds71 ==
  In1 : Inport
  Assumption : sldvlib/Objectives and Constraints/Assumption  enabled=on  customAVTBlockType=Assumption  intervals=true  initial=off  dispValues=on  outEnabled=on
      settings: AttributesFormatString=%<intervals>
  Logical Operator : Logic  AllPortsSameDT=off  OutDataTypeStr=boolean
  geq : RelationalOperator  Operator=<=  OutDataTypeStr=boolean
  lb : Constant  OutDataTypeStr=int8
  leq : RelationalOperator  Operator=<=  OutDataTypeStr=boolean  InputSameDT=on
  ub : Constant  Value=9  OutDataTypeStr=int8
  wires:
  In1/1 -> geq/1, leq/2
  geq/1 -> Logical Operator/2
  ub/1 -> geq/2
  leq/1 -> Logical Operator/1
  Logical Operator/1 -> Assumption/1
  lb/1 -> leq/1

== system sudoku/bounds72 ==
  In1 : Inport
  Assumption : sldvlib/Objectives and Constraints/Assumption  enabled=on  customAVTBlockType=Assumption  intervals=true  initial=off  dispValues=on  outEnabled=on
      settings: AttributesFormatString=%<intervals>
  Logical Operator : Logic  AllPortsSameDT=off  OutDataTypeStr=boolean
  geq : RelationalOperator  Operator=<=  OutDataTypeStr=boolean
  lb : Constant  OutDataTypeStr=int8
  leq : RelationalOperator  Operator=<=  OutDataTypeStr=boolean  InputSameDT=on
  ub : Constant  Value=9  OutDataTypeStr=int8
  wires:
  In1/1 -> geq/1, leq/2
  geq/1 -> Logical Operator/2
  ub/1 -> geq/2
  leq/1 -> Logical Operator/1
  Logical Operator/1 -> Assumption/1
  lb/1 -> leq/1

== system sudoku/bounds73 ==
  In1 : Inport
  Assumption : sldvlib/Objectives and Constraints/Assumption  enabled=on  customAVTBlockType=Assumption  intervals=true  initial=off  dispValues=on  outEnabled=on
      settings: AttributesFormatString=%<intervals>
  Logical Operator : Logic  AllPortsSameDT=off  OutDataTypeStr=boolean
  geq : RelationalOperator  Operator=<=  OutDataTypeStr=boolean
  lb : Constant  OutDataTypeStr=int8
  leq : RelationalOperator  Operator=<=  OutDataTypeStr=boolean  InputSameDT=on
  ub : Constant  Value=9  OutDataTypeStr=int8
  wires:
  In1/1 -> geq/1, leq/2
  geq/1 -> Logical Operator/2
  ub/1 -> geq/2
  leq/1 -> Logical Operator/1
  Logical Operator/1 -> Assumption/1
  lb/1 -> leq/1

== system sudoku/bounds74 ==
  In1 : Inport
  Assumption : sldvlib/Objectives and Constraints/Assumption  enabled=on  customAVTBlockType=Assumption  intervals=true  initial=off  dispValues=on  outEnabled=on
      settings: AttributesFormatString=%<intervals>
  Logical Operator : Logic  AllPortsSameDT=off  OutDataTypeStr=boolean
  geq : RelationalOperator  Operator=<=  OutDataTypeStr=boolean
  lb : Constant  OutDataTypeStr=int8
  leq : RelationalOperator  Operator=<=  OutDataTypeStr=boolean  InputSameDT=on
  ub : Constant  Value=9  OutDataTypeStr=int8
  wires:
  In1/1 -> geq/1, leq/2
  geq/1 -> Logical Operator/2
  ub/1 -> geq/2
  leq/1 -> Logical Operator/1
  Logical Operator/1 -> Assumption/1
  lb/1 -> leq/1

== system sudoku/bounds75 ==
  In1 : Inport
  Assumption : sldvlib/Objectives and Constraints/Assumption  enabled=on  customAVTBlockType=Assumption  intervals=true  initial=off  dispValues=on  outEnabled=on
      settings: AttributesFormatString=%<intervals>
  Logical Operator : Logic  AllPortsSameDT=off  OutDataTypeStr=boolean
  geq : RelationalOperator  Operator=<=  OutDataTypeStr=boolean
  lb : Constant  OutDataTypeStr=int8
  leq : RelationalOperator  Operator=<=  OutDataTypeStr=boolean  InputSameDT=on
  ub : Constant  Value=9  OutDataTypeStr=int8
  wires:
  In1/1 -> geq/1, leq/2
  geq/1 -> Logical Operator/2
  ub/1 -> geq/2
  leq/1 -> Logical Operator/1
  Logical Operator/1 -> Assumption/1
  lb/1 -> leq/1

== system sudoku/bounds76 ==
  In1 : Inport
  Assumption : sldvlib/Objectives and Constraints/Assumption  enabled=on  customAVTBlockType=Assumption  intervals=true  initial=off  dispValues=on  outEnabled=on
      settings: AttributesFormatString=%<intervals>
  Logical Operator : Logic  AllPortsSameDT=off  OutDataTypeStr=boolean
  geq : RelationalOperator  Operator=<=  OutDataTypeStr=boolean
  lb : Constant  OutDataTypeStr=int8
  leq : RelationalOperator  Operator=<=  OutDataTypeStr=boolean  InputSameDT=on
  ub : Constant  Value=9  OutDataTypeStr=int8
  wires:
  In1/1 -> geq/1, leq/2
  geq/1 -> Logical Operator/2
  ub/1 -> geq/2
  leq/1 -> Logical Operator/1
  Logical Operator/1 -> Assumption/1
  lb/1 -> leq/1

== system sudoku/bounds77 ==
  In1 : Inport
  Assumption : sldvlib/Objectives and Constraints/Assumption  enabled=on  customAVTBlockType=Assumption  intervals=true  initial=off  dispValues=on  outEnabled=on
      settings: AttributesFormatString=%<intervals>
  Logical Operator : Logic  AllPortsSameDT=off  OutDataTypeStr=boolean
  geq : RelationalOperator  Operator=<=  OutDataTypeStr=boolean
  lb : Constant  OutDataTypeStr=int8
  leq : RelationalOperator  Operator=<=  OutDataTypeStr=boolean  InputSameDT=on
  ub : Constant  Value=9  OutDataTypeStr=int8
  wires:
  In1/1 -> geq/1, leq/2
  geq/1 -> Logical Operator/2
  ub/1 -> geq/2
  leq/1 -> Logical Operator/1
  Logical Operator/1 -> Assumption/1
  lb/1 -> leq/1

== system sudoku/bounds78 ==
  In1 : Inport
  Assumption : sldvlib/Objectives and Constraints/Assumption  enabled=on  customAVTBlockType=Assumption  intervals=true  initial=off  dispValues=on  outEnabled=on
      settings: AttributesFormatString=%<intervals>
  Logical Operator : Logic  AllPortsSameDT=off  OutDataTypeStr=boolean
  geq : RelationalOperator  Operator=<=  OutDataTypeStr=boolean
  lb : Constant  OutDataTypeStr=int8
  leq : RelationalOperator  Operator=<=  OutDataTypeStr=boolean  InputSameDT=on
  ub : Constant  Value=9  OutDataTypeStr=int8
  wires:
  In1/1 -> geq/1, leq/2
  geq/1 -> Logical Operator/2
  ub/1 -> geq/2
  leq/1 -> Logical Operator/1
  Logical Operator/1 -> Assumption/1
  lb/1 -> leq/1

== system sudoku/bounds79 ==
  In1 : Inport
  Assumption : sldvlib/Objectives and Constraints/Assumption  enabled=on  customAVTBlockType=Assumption  intervals=true  initial=off  dispValues=on  outEnabled=on
      settings: AttributesFormatString=%<intervals>
  Logical Operator : Logic  AllPortsSameDT=off  OutDataTypeStr=boolean
  geq : RelationalOperator  Operator=<=  OutDataTypeStr=boolean
  lb : Constant  OutDataTypeStr=int8
  leq : RelationalOperator  Operator=<=  OutDataTypeStr=boolean  InputSameDT=on
  ub : Constant  Value=9  OutDataTypeStr=int8
  wires:
  In1/1 -> geq/1, leq/2
  geq/1 -> Logical Operator/2
  ub/1 -> geq/2
  leq/1 -> Logical Operator/1
  Logical Operator/1 -> Assumption/1
  lb/1 -> leq/1

== system sudoku/bounds8 ==
  In1 : Inport
  Assumption : sldvlib/Objectives and Constraints/Assumption  enabled=on  customAVTBlockType=Assumption  intervals=true  initial=off  dispValues=on  outEnabled=on
      settings: AttributesFormatString=%<intervals>
  Logical Operator : Logic  AllPortsSameDT=off  OutDataTypeStr=boolean
  geq : RelationalOperator  Operator=<=  OutDataTypeStr=boolean
  lb : Constant  OutDataTypeStr=int8
  leq : RelationalOperator  Operator=<=  OutDataTypeStr=boolean
  ub : Constant  Value=9  OutDataTypeStr=int8
  wires:
  In1/1 -> geq/1, leq/2
  geq/1 -> Logical Operator/2
  ub/1 -> geq/2
  leq/1 -> Logical Operator/1
  Logical Operator/1 -> Assumption/1
  lb/1 -> leq/1

== system sudoku/bounds80 ==
  In1 : Inport
  Assumption : sldvlib/Objectives and Constraints/Assumption  enabled=on  customAVTBlockType=Assumption  intervals=true  initial=off  dispValues=on  outEnabled=on
      settings: AttributesFormatString=%<intervals>
  Logical Operator : Logic  AllPortsSameDT=off  OutDataTypeStr=boolean
  geq : RelationalOperator  Operator=<=  OutDataTypeStr=boolean
  lb : Constant  OutDataTypeStr=int8
  leq : RelationalOperator  Operator=<=  OutDataTypeStr=boolean  InputSameDT=on
  ub : Constant  Value=9  OutDataTypeStr=int8
  wires:
  In1/1 -> geq/1, leq/2
  geq/1 -> Logical Operator/2
  ub/1 -> geq/2
  leq/1 -> Logical Operator/1
  Logical Operator/1 -> Assumption/1
  lb/1 -> leq/1

== system sudoku/bounds81 ==
  In1 : Inport
  Assumption : sldvlib/Objectives and Constraints/Assumption  enabled=on  customAVTBlockType=Assumption  intervals=true  initial=off  dispValues=on  outEnabled=on
      settings: AttributesFormatString=%<intervals>
  Logical Operator : Logic  AllPortsSameDT=off  OutDataTypeStr=boolean
  geq : RelationalOperator  Operator=<=  OutDataTypeStr=boolean
  lb : Constant  OutDataTypeStr=int8
  leq : RelationalOperator  Operator=<=  OutDataTypeStr=boolean  InputSameDT=on
  ub : Constant  Value=9  OutDataTypeStr=int8
  wires:
  In1/1 -> geq/1, leq/2
  geq/1 -> Logical Operator/2
  ub/1 -> geq/2
  leq/1 -> Logical Operator/1
  Logical Operator/1 -> Assumption/1
  lb/1 -> leq/1
